simulink library "quat_smoother"  (R2018b)
settings: Solver=VariableStepAuto  StartTime=0.0  StopTime=10.0  RelTol=1e-3
undefined symbols (not defined in the file or in its folder): fswParams
libraries: aerolibutil x2, quat_rectify_lib x1
settings Model: Creator=Nick's PC  LastModifiedBy=Nick's PC

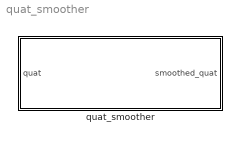
== system quat_smoother ==
  quat_smoother : Subsystem

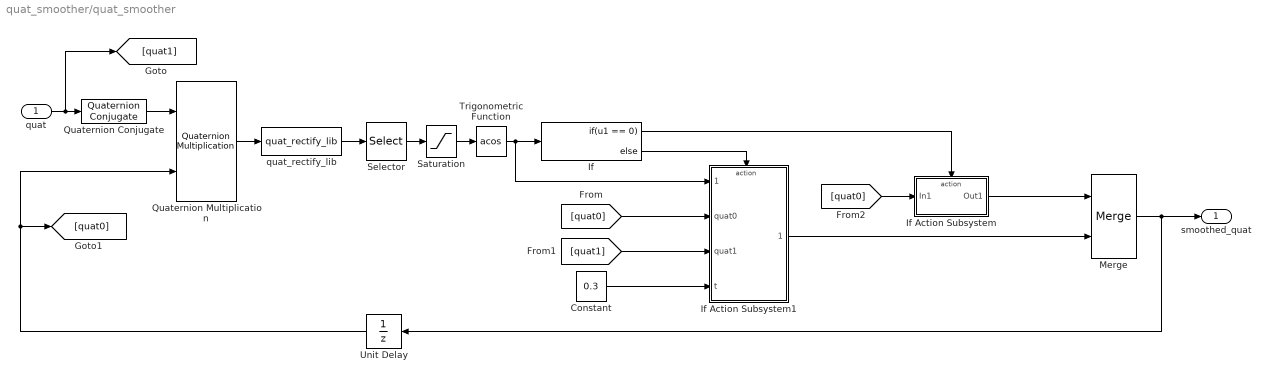
== system quat_smoother/quat_smoother ==
  quat : Inport
  Constant : Constant  Value=0.3
  If : If  IfExpression=u1 == 0
  If Action Subsystem : Subsystem  TreatAsAtomicUnit=on
  If Action Subsystem1 : Subsystem  TreatAsAtomicUnit=on
  Merge : Merge
  Quaternion Conjugate : aerolibutil/Quaternion Conjugate
      settings: SourceProductName=Aerospace Blockset  SourceProductBaseCode=AE
  Quaternion Multiplication : aerolibutil/Quaternion Multiplication
  Saturation : Saturate  UpperLimit=1  LowerLimit=-1
  Selector : Selector  InputPortWidth=4  IndexOptions=Index vector (dialog)  Indices=1  OutputSizes=1
  Trigonometric Function : Trigonometry  Operator=acos
  Unit Delay : UnitDelay  InitialCondition=fswParams.estimation.ic.quat_est_init  SampleTime=fswParams.sample_time_s
  quat_rectify_lib : quat_rectify_lib/quat_rectify_lib
  smoothed_quat : Outport
  wires:
  Unit Delay/1 -> Quaternion Multiplication/2, [quat0]
  Trigonometric Function/1 -> If Action Subsystem1/1(rad_err_2), If/1
  Saturation/1 -> Trigonometric Function/1
  quat_rectify_lib/1 -> Selector/1
  Quaternion Multiplication/1 -> quat_rectify_lib/1
  Selector/1 -> Saturation/1
  Quaternion Conjugate/1 -> Quaternion Multiplication/1
  quat/1 -> [quat1], Quaternion Conjugate/1
  If/1 -> If Action Subsystem/Action
  If/2 -> If Action Subsystem1/Action
  [quat0] -> If Action Subsystem1/2(quat0)
  [quat1] -> If Action Subsystem1/3(quat1)
  [quat0] -> If Action Subsystem/1(In1)
  Constant/1 -> If Action Subsystem1/4(t)
  If Action Subsystem/1(Out1) -> Merge/1
  If Action Subsystem1/1(smoothed_quat) -> Merge/2
  Merge/1 -> Unit Delay/1, smoothed_quat/1

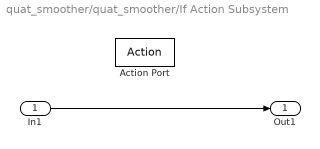
== system quat_smoother/quat_smoother/If Action Subsystem ==
  In1 : Inport
  Action Port : ActionPort  ActionType=then
  Out1 : Outport
  wires:
  In1/1 -> Out1/1

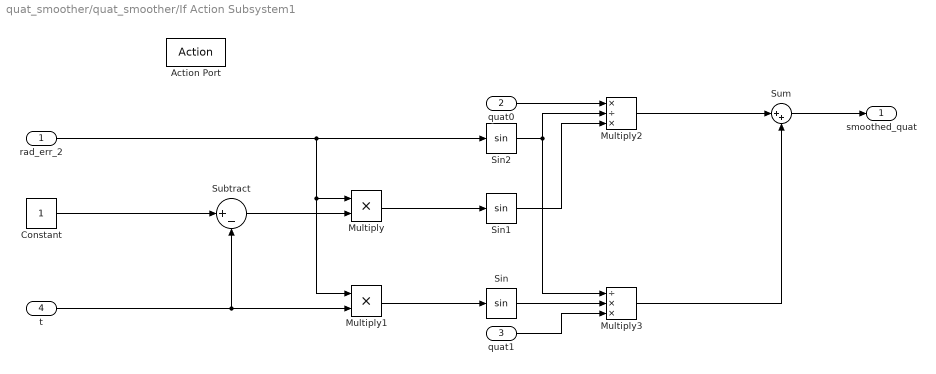
== system quat_smoother/quat_smoother/If Action Subsystem1 ==
  rad_err_2 : Inport
  quat0 : Inport  Port=2
  quat1 : Inport  Port=3
  t : Inport  Port=4
  Action Port : ActionPort  ActionType=else
  Constant : Constant
  Multiply : Product
  Multiply1 : Product
  Multiply2 : Product  Inputs=*/*
  Multiply3 : Product  Inputs=/**
  Sin : Trigonometry
  Sin1 : Trigonometry
  Sin2 : Trigonometry
  Subtract : Sum  Inputs=|+-
  Sum : Sum  Inputs=|++
  smoothed_quat : Outport
  wires:
  Constant/1 -> Subtract/1
  t/1 -> Multiply1/2, Subtract/2
  rad_err_2/1 -> Sin2/1, Multiply1/1, Multiply/1
  Subtract/1 -> Multiply/2
  Multiply1/1 -> Sin/1
  Multiply/1 -> Sin1/1
  quat0/1 -> Multiply2/1
  Sin2/1 -> Multiply3/1, Multiply2/2
  Sin1/1 -> Multiply2/3
  Sin/1 -> Multiply3/2
  quat1/1 -> Multiply3/3
  Multiply3/1 -> Sum/2
  Multiply2/1 -> Sum/1
  Sum/1 -> smoothed_quat/1
